simulink model "PR_1_var2"  (R2020b)
settings: Solver=VariableStepAuto  StartTime=0.0  StopTime=10  RelTol=1e-3
settings Model: Creator=SIA  LastModifiedBy=SIA

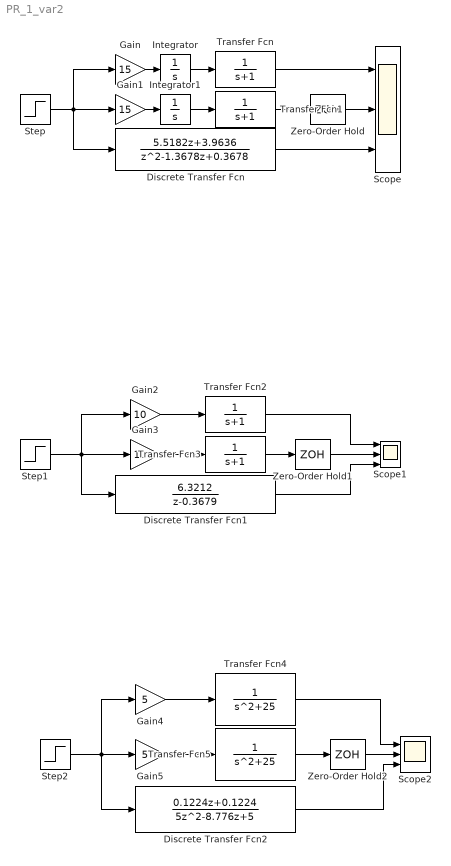
== system PR_1_var2 ==
  Discrete Transfer Fcn : DiscreteTransferFcn  Numerator=[5.5182 3.9636]  Denominator=[1 -1.3678 0.3678]  SampleTime=1
  Discrete Transfer Fcn1 : DiscreteTransferFcn  Numerator=[6.3212]  Denominator=[1 -0.3679]  SampleTime=1
  Discrete Transfer Fcn2 : DiscreteTransferFcn  Numerator=[0.1224 0.1224]  Denominator=[5 -8.776 5]
  Gain : Gain  Gain=15
  Gain1 : Gain  Gain=15
  Gain2 : Gain  Gain=10
  Gain3 : Gain  Gain=10
  Gain4 : Gain  Gain=5
  Gain5 : Gain  Gain=5
  Integrator : Integrator
  Integrator1 : Integrator
  Scope : Scope  NumInputPorts=3
  Scope1 : Scope  NumInputPorts=3
  Scope2 : Scope  NumInputPorts=3
  Step : Step  Time=0
  Step1 : Step  Time=0  SampleTime=0
  Step2 : Step  Time=0  SampleTime=0
  Transfer Fcn{,1..3} (4 alike) : TransferFcn  Denominator=[1 1]
  Transfer Fcn4 : TransferFcn  Denominator=[1 0 25]
  Transfer Fcn5 : TransferFcn  Denominator=[1 0 25]
  Zero-Order Hold : ZeroOrderHold
  Zero-Order Hold1 : ZeroOrderHold
  Zero-Order Hold2 : ZeroOrderHold  SampleTime=0.1
  wires:
  Step/1 -> Gain/1, Discrete Transfer Fcn/1, Gain1/1
  Discrete Transfer Fcn/1 -> Scope/3
  Zero-Order Hold/1 -> Scope/2
  Transfer Fcn/1 -> Scope/1
  Transfer Fcn1/1 -> Zero-Order Hold/1
  Integrator1/1 -> Transfer Fcn1/1
  Integrator/1 -> Transfer Fcn/1
  Gain/1 -> Integrator/1
  Gain1/1 -> Integrator1/1
  Transfer Fcn2/1 -> Scope1/1
  Zero-Order Hold1/1 -> Scope1/2
  Gain3/1 -> Transfer Fcn3/1
  Transfer Fcn3/1 -> Zero-Order Hold1/1
  Step1/1 -> Discrete Transfer Fcn1/1, Gain2/1, Gain3/1
  Gain2/1 -> Transfer Fcn2/1
  Discrete Transfer Fcn1/1 -> Scope1/3
  Step2/1 -> Gain4/1, Discrete Transfer Fcn2/1, Gain5/1
  Transfer Fcn5/1 -> Zero-Order Hold2/1
  Zero-Order Hold2/1 -> Scope2/2
  Discrete Transfer Fcn2/1 -> Scope2/3
  Transfer Fcn4/1 -> Scope2/1
  Gain5/1 -> Transfer Fcn5/1
  Gain4/1 -> Transfer Fcn4/1
